simulink model "Model3D_PY"  (R2020a)
settings: Solver=ode15s  StartTime=0.0  StopTime=100  RelTol=1e-3
model workspace (MAT data in the model file):
  VEH : object (value not decoded)
  color : object (value not decoded)
  cosAngle = 1
  density : object (value not decoded)
  dwb : object (value not decoded)
  mp : object (value not decoded)
  number1 = 5
  platform : object (value not decoded)
  pr : object (value not decoded)
  sinAngle = 1
  wheel : object (value not decoded)
undefined symbols (not defined in the file or in its folder): f
libraries: autolibutils x4, sim3dlib x3, autolibshared x2, simulink x1, vdynlib x1, vehdynlibsteering x1, instrumentlib x1
(part 3 of 3)

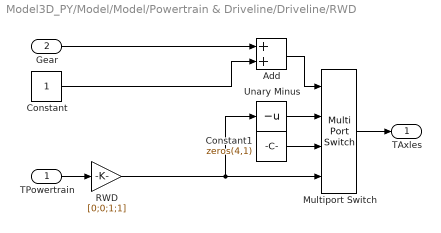
== system Model3D_PY/Model/Model/Powertrain & Driveline/Driveline/RWD ==
  TPowertrain : Inport
  Gear : Inport  Port=2
  Add : Sum
  Constant : Constant
  Constant1 : Constant  Value=zeros(4,1)
  Multiport Switch : MultiPortSwitch  DataPortOrder=Zero-based contiguous  zeroidx=on
  RWD : Gain  Gain=[0;0;1;1]
  Unary Minus : UnaryMinus
  TAxles : Outport  VectorParamsAs1DForOutWhenUnconnected=off
  wires:
  RWD/1 -> Unary Minus/1, Multiport Switch/4
  TPowertrain/1 -> RWD/1
  Unary Minus/1 -> Multiport Switch/2
  Multiport Switch/1 -> TAxles/1
  Gear/1 -> Add/1
  Constant/1 -> Add/2
  Add/1 -> Multiport Switch/1
  Constant1/1 -> Multiport Switch/3
